simulink model "A2_7_P_angle_ramp"  (Simulink 7.4)
settings: Solver=FixedStepDiscrete  StartTime=0.0  StopTime=10  RelTol=1e-3
undefined symbols (not defined in the file): Kp
libraries: simulink x1, DCmotor_library x1
settings Model: Creator=Natalia  LastModifiedBy=ma
settings DebuggingCC: StrictBusMsg=ErrorLevel1
settings HardwareCC: ProdIntDivRoundTo=Zero  ProdEndianess=LittleEndian  ProdHWDeviceType=Generic->32-bit x86 compatible
settings RTWCC: SystemTargetFile=rtwin.tlc  TemplateMakefile=rtwin.tmf  Description=Real-Time Windows Target  ProcessScript=rtwin_make_rtw_hook  RTWCompilerOptimization=On
settings CodeAppCC: MaxIdLength=95  CustomSymbolStrType=$N$R$M_T
settings TargetCC: TargetLibSuffix=_rtwin.lib  TargetPreCompLibLocation=C:\Program Files\MATLAB\R2012b\toolbox\rtw\targets\rtwin\lib\win64  TargetFunctionLibrary=ANSI_C  IsPILTarget=off  MatFileLogging=on  EnableShiftOperators=on
settings CustomProperty: DataType=string  Value=C:/PROGRA~1/MATLAB/R2012b/toolbox/rtw/targets/rtwin

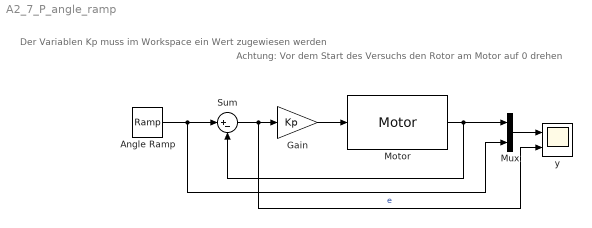
== system A2_7_P_angle_ramp ==
  note: Achtung:
      | Vor dem Start des Versuchs
      | den Rotor am Motor auf 0 drehen
  note: Der Variablen
      | Kp muss im Workspace ein
      | Wert zugewiesen werden
  Angle Ramp : simulink/Sources/Ramp  slope=20  start=1  X0=0
  Gain : Gain  Gain=Kp
  Motor : DCmotor_library/Motor  motoridinput=1  name_signal=Angle  ts=10
  Mux : Mux  Inputs=2
  Sum : Sum  Inputs=|+-
  y : Scope  NumInputPorts=2
      settings: YMin=-10~-7  YMax=140~8  SaveName=ScopeData2
  wires:
  Angle Ramp/1 -> Mux/2, Sum/1
  Sum/1 -> y/2, Gain/1  "e"
  Motor/1 -> Mux/1, Sum/2
  Mux/1 -> y/1
  Gain/1 -> Motor/1
